simulink model "pendule_model"  (R2025b)
settings: Solver=VariableStepAuto  StartTime=0.0  StopTime=6  RelTol=1e-3
undefined symbols (not defined in the file): A, B, C, C_obs, dq0, H_cmd, K_cmd, L_obs, q0
settings Model: Creator=victor  LastModifiedBy=victor

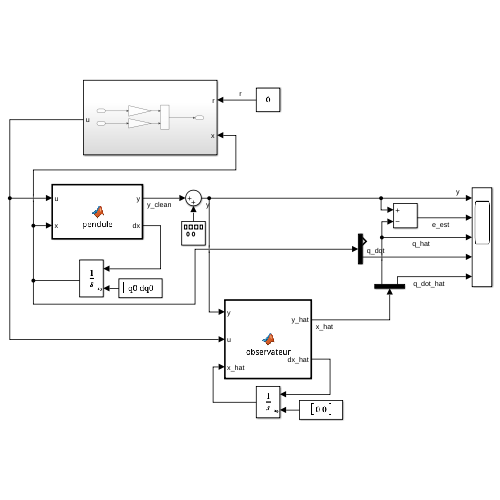
[thumbnail: Simulink's stored preview of the top-level diagram]
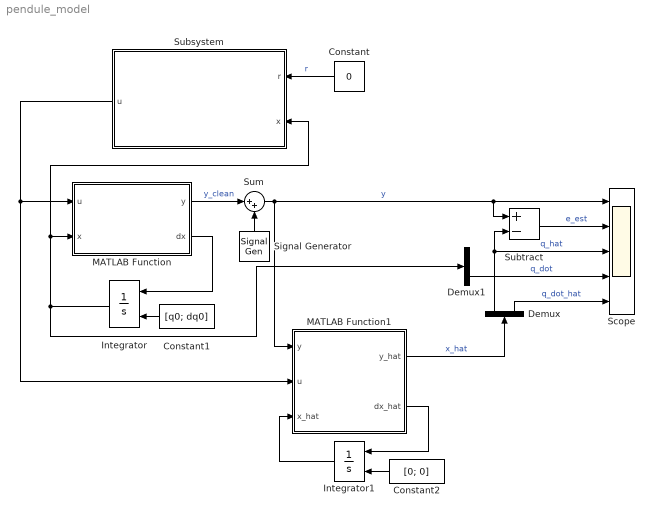
== system pendule_model ==
  Constant : Constant  Value=0
  Constant1 : Constant  Value=[q0; dq0]
  Constant2 : Constant  Value=[0; 0]
  Demux : Demux  Outputs=2
  Demux1 : Demux  Outputs=2
  Integrator : Integrator  InitialConditionSource=external
  Integrator1 : Integrator  InitialConditionSource=external
  MATLAB Function : MATLAB Function  TreatAsAtomicUnit=on
  MATLAB Function1 : MATLAB Function  TreatAsAtomicUnit=on
  Scope : Scope  NumInputPorts=5
      settings: ActiveDisplayYMinimum=-0.35180674711943061  ActiveDisplayYMaximum=0.52630878390345393
  Signal Generator : SignalGenerator  Amplitude=0.01  Frequency=100  Units=rad/sec
  Subsystem : Subsystem
  Subtract : Sum  Inputs=+-
  Sum : Sum  Inputs=|++
  wires:
  Sum/1 -> Subtract/1, Scope/1, MATLAB Function1/1(y)  "y"
  MATLAB Function/2(dx) -> Integrator/1
  Integrator/1 -> Subsystem/2(x), MATLAB Function/2(x), Demux1/1
  MATLAB Function1/2(dx_hat) -> Integrator1/1
  Integrator1/1 -> MATLAB Function1/3(x_hat)
  MATLAB Function1/1(y_hat) -> Demux/1  "x_hat"
  Subtract/1 -> Scope/2  "e_est"
  Constant1/1 -> Integrator/2
  Demux/1 -> Subtract/2, Scope/3  "q_hat"
  Demux/2 -> Scope/5  "q_dot_hat"
  Demux1/2 -> Scope/4  "q_dot"
  Constant2/1 -> Integrator1/2
  Subsystem/1(u) -> MATLAB Function/1(u), MATLAB Function1/2(u)
  Constant/1 -> Subsystem/1(r)  "r"
  Signal Generator/1 -> Sum/2
  MATLAB Function/1(y) -> Sum/1  "y_clean"

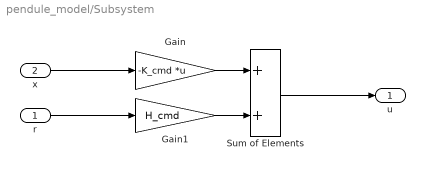
== system pendule_model/Subsystem ==
  r : Inport
  x : Inport  Port=2
  Gain : Gain  Gain=-K_cmd  Multiplication=Matrix(K*u)
  Gain1 : Gain  Gain=H_cmd
  Sum of Elements : Sum
  u : Outport
  wires:
  Gain1/1 -> Sum of Elements/2
  r/1 -> Gain1/1
  Gain/1 -> Sum of Elements/1
  Sum of Elements/1 -> u/1
  x/1 -> Gain/1

== matlab function pendule_model/MATLAB Function1 ==
  data: y input; u input; y_hat output; x_hat input; dx_hat output; A parameter; B parameter; C_obs parameter; L_obs parameter; C parameter
function [y_hat, dx_hat] = observateur(y, u, x_hat, A, B, C_obs, L_obs, C)
dx_hat = zeros(2, 1);
dx_hat = A*x_hat + B*u + L_obs*(y - C*x_hat);
y_hat = C_obs*x_hat;

== matlab function pendule_model/MATLAB Function ==
  data: u input; y output; x input; dx output; A parameter; B parameter; C parameter
function [y, dx] = pendule(u, x, A, B, C)
dx = zeros(2, 1);
dx = A*x + B*u;
y = C*x;
